simulink model "VTD_PLL"  (R2024b)
settings: Solver=VariableStepAuto  StartTime=0.0  StopTime=0.5  RelTol=1e-3
undefined symbols (not defined in the file): DiscIntNeverNeededParam, dspblkCoreblockFVToolHelper, gcbh
libraries: slpidlib x1
settings Model: Creator=byrin  LastModifiedBy=byrin

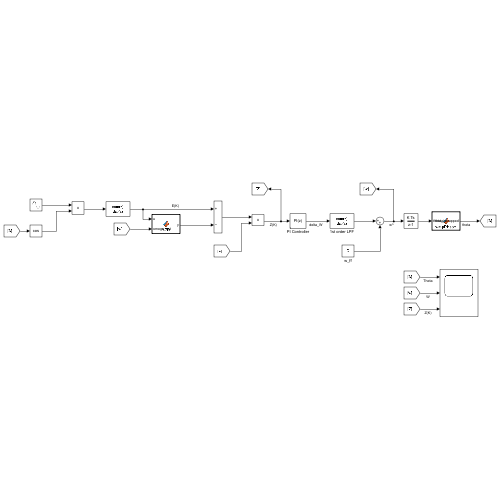
[thumbnail: Simulink's stored preview of the top-level diagram]
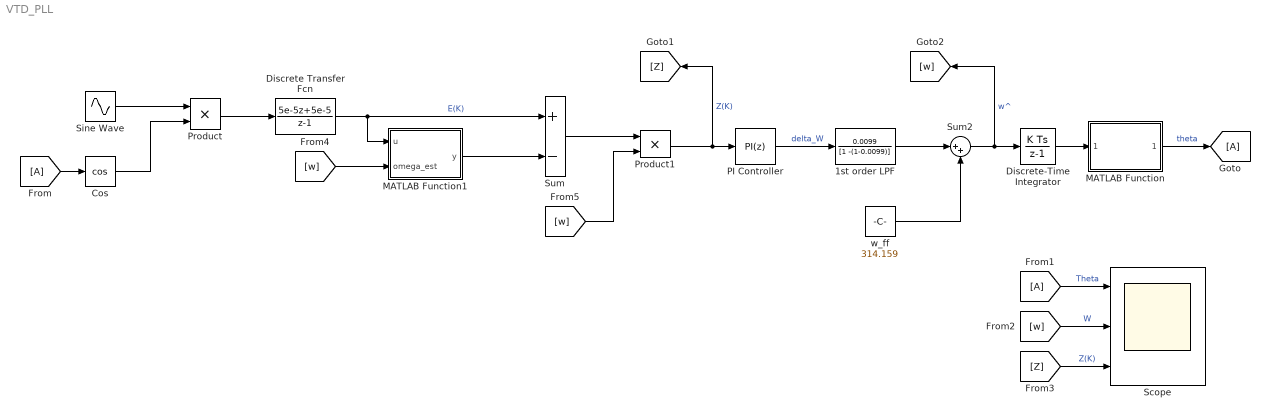
== system VTD_PLL ==
  1st order LPF : DiscreteTransferFcn  LoadFcn=dspblkCoreblockFVToolHelper(gcbh,'load');  Numerator=[0.0099]  Denominator=[1 -(1-0.0099)]
      settings: CopyFcn=dspblkCoreblockFVToolHelper(gcbh,'copy');  DeleteFcn=dspblkCoreblockFVToolHelper(gcbh,'close');  ModelCloseFcn=dspblkCoreblockFVToolHelper(gcbh,'close');  PreSaveFcn=dspblkCoreblockFVToolHelper(gcbh,'presave');  PostSaveFcn=dspblkCoreblockFVToolHelper(gcbh,'postsave');  CloseFcn=dspblkCoreblockFVToolHelper(gcbh,'close');
  Cos : Trigonometry  Operator=cos
  Discrete Transfer Fcn : DiscreteTransferFcn  LoadFcn=dspblkCoreblockFVToolHelper(gcbh,'load');  Numerator=[5e-5 5e-5]  Denominator=[1 -1]
      settings: CopyFcn=dspblkCoreblockFVToolHelper(gcbh,'copy');  DeleteFcn=dspblkCoreblockFVToolHelper(gcbh,'close');  ModelCloseFcn=dspblkCoreblockFVToolHelper(gcbh,'close');  PreSaveFcn=dspblkCoreblockFVToolHelper(gcbh,'presave');  PostSaveFcn=dspblkCoreblockFVToolHelper(gcbh,'postsave');  CloseFcn=dspblkCoreblockFVToolHelper(gcbh,'close');
  Discrete-Time Integrator : DiscreteIntegrator  SampleTime=1e-4  ICPrevOutput=DiscIntNeverNeededParam  ICPrevScaledInput=DiscIntNeverNeededParam
  From : From
  From1 : From
  Goto : Goto
  MATLAB Function : MATLAB Function  TreatAsAtomicUnit=on
  MATLAB Function1 : MATLAB Function  TreatAsAtomicUnit=on
  PI Controller : slpidlib/PID Controller  Controller=PI  Form=Parallel  TimeDomain=Discrete-time  UseExternalTs=off  SampleTime=1e-4  IntegratorMethod=Forward Euler  FilterMethod=Forward Euler  ControllerParametersSource=internal  P=104  I=4521  UseKiTs=off  D=0  UseExternalDerivativeSource=off  N=100  UseFilter=on  TunerSelectOption=Transfer Function Based (PID Tuner App)  InitialConditionSource=internal  InitialConditionForIntegrator=0  InitialConditionForFilter=0  DifferentiatorICPrevScaledInput=0  ExternalReset=none  TrackingMode=off  Kt=1  LimitOutput=off  SatLimitsSource=internal  UpperSaturationLimit=inf  LowerSaturationLimit=-inf  LinearizeAsGain=on  AntiWindupMode=none  Kb=1  LimitIntegrator=off  UpperIntegratorSaturationLimit=inf  LowerIntegratorSaturationLimit=-inf  POutMin=[]  POutMax=[]  IOutMin=[]  IOutMax=[]  DOutMin=[]  DOutMax=[]  NOutMin=[]  NOutMax=[]  SumOutMin=[]  SumOutMax=[]  SaturationOutMin=[]  SaturationOutMax=[]  PParamMin=[]  PParamMax=[]  IParamMin=[]  IParamMax=[]  DParamMin=[]  DParamMax=[]  NParamMin=[]  NParamMax=[]  KbParamMin=[]  KbParamMax=[]  KtParamMin=[]  KtParamMax=[]  KbOutMin=[]  KbOutMax=[]  KtOutMin=[]  KtOutMax=[]  IntegratorOutMin=[]  IntegratorOutMax=[]  FilterOutMin=[]  FilterOutMax=[]  SumI1OutMin=[]  SumI1OutMax=[]  SumI2OutMin=[]  SumI2OutMax=[]  SumI3OutMin=[]  SumI3OutMax=[]  SumI4OutMin=[]  SumI4OutMax=[]  SumDOutMin=[]  SumDOutMax=[]  DifferentiatorOutMin=[]  DifferentiatorOutMax=[]  FilterDiffOutCoefMin=[]  FilterDiffOutCoefMax=[]  ReciprocalOutMin=[]  ReciprocalOutMax=[]  SumDenOutMin=[]  SumDenOutMax=[]  SumNumOutMin=[]  SumNumOutMax=[]  DivideOutMin=[]  DivideOutMax=[]  UdiffTsProdOutMin=[]  UdiffTsProdOutMax=[]  NTsProdOutMin=[]  NTsProdOutMax=[]  UintegralTsProdOutMin=[]  UintegralTsProdOutMax=[]  UngainTsProdOutMin=[]  UngainTsProdOutMax=[]  ClampingZeroOutDataTypeStr=Inherit: Inherit via back propagation  ClampingZeroOutMin=[]  ClampingZeroOutMax=[]  FilterDenConstantOutDataTypeStr=Inherit: Inherit via back propagation  FilterDenConstantOutMin=[]  FilterDenConstantOutMax=[]  PCopyOutDataTypeStr=Inherit: Inherit via back propagation  PCopyOutMin=[]  PCopyOutMax=[]  NCopyOutDataTypeStr=Inherit: Inherit via back propagation  NCopyOutMin=[]  NCopyOutMax=[]  IntegratorContinuousStateAttributes=''  IntegratorStateMustResolveToSignalObject=off  IntegratorRTWStateStorageClass=Auto  FilterContinuousStateAttributes=''  FilterStateMustResolveToSignalObject=off  FilterRTWStateStorageClass=Auto  ParallelPVariant=InternalParameters  IdealPVariant=Disabled  IVariant=InternalParameters  DVariant=Disabled  IntegratorVariant=Discrete  SatVariant=Disabled  AWVariant=Passthrough  PCopyVariant=Disabled  TRVariant=Disabled  FdbkBlocksVariant=Forward  IdealPFdbkVariant=Disabled  SatFdbkVariant=Disabled  DerivativeFilterVariant=Disabled  NVariant=Disabled  NCopyVariant=Disabled_SignalSpec  FilterICVariant=Disabled  IntegratorICVariant=InternalICs  ExternalResetVariant=Disabled  TRSumVariant=Passthrough  SumFdbkVariant=Disabled  SumVariant=Sum_PI  TsampFilterVariant=InternalTs  TsampNgainVariant=Passthrough  TsampIntegralVariant=Disabled_SignalSpec  ExternalSaturationOutDataTypeStr=Inherit: Same as second input  DerivativeSourceVariant=Disabled  PreIntVariant=InternalPreInt
  Product : Product
  Product1 : Product
  Scope : Scope  NumInputPorts=3
  Sine Wave : Sin  Frequency=50  SampleTime=1e-4
  Sum : Sum  Inputs=+-
  Sum2 : Sum  Inputs=|++
  w_ff : Constant  Value=314.159
  wires:
  MATLAB Function/1(theta_wrapped) -> Goto/1  "theta"
  Sum2/1 -> [w], Discrete-Time Integrator/1  "w^"
  1st order LPF/1 -> Sum2/1
  w_ff/1 -> Sum2/2
  PI Controller/1 -> 1st order LPF/1  "delta_W"
  Discrete-Time Integrator/1 -> MATLAB Function/1(theta_in)
  Product1/1 -> [Z], PI Controller/1  "Z(K)"
  Sine Wave/1 -> Product/1
  From/1 -> Cos/1
  Cos/1 -> Product/2
  Discrete Transfer Fcn/1 -> MATLAB Function1/1(u), Sum/1  "E(K)"
  MATLAB Function1/1(y) -> Sum/2
  Product/1 -> Discrete Transfer Fcn/1
  Sum/1 -> Product1/1
  From1/1 -> Scope/1  "Theta"
  [w] -> Scope/2  "W"
  [Z] -> Scope/3  "Z(K)"
  [w] -> MATLAB Function1/2(omega_est)
  [w] -> Product1/2

== matlab function VTD_PLL/MATLAB Function ==
  data: theta_in input; theta_wrapped output
function theta_wrapped = wrapPhase(theta_in)
% Wraps phase to [0, 2*pi)
theta_wrapped = mod(theta_in, 2*pi);
end

== matlab function VTD_PLL/MATLAB Function1 ==
  data: u input; y output; omega_est input
function y = VTD(u, omega_est)
% --- PARAMETERS ---
fs = 1e4;             % Sampling frequency (Hz) -> Ts=1e-4
maxDelay = 2000;      % Max buffer length for safety (~0.2 s at fs=10kHz)

% --- PERSISTENT BUFFER ---
persistent buffer idx
if isempty(buffer)
    buffer = zeros(1, maxDelay);
    idx = 1;
end

% --- Compute delay length ---
% Convert omega (rad/s) to frequency in Hz
f_est = omega_est / (2*pi);
if f_est < 1
    f_est = 1;  % avoid division by zero for very small freq
end
% Quarter cycle delay length in samples
N = round(fs / (4*f_est));

% --- Store new sample ---
buffer(idx) = u;

% --- Delayed index ---
delay_idx = mod(idx - N - 1, maxDelay) + 1;
y = buffer(delay_idx);

% --- Update pointer ---
idx = mod(idx, maxDelay) + 1;
end
